simulink model "openloop5012"  (R2022a)
settings: Solver=VariableStepAuto  StartTime=0.0  StopTime=5000  RelTol=1e-3
settings Model: Creator=danie  LastModifiedBy=danie

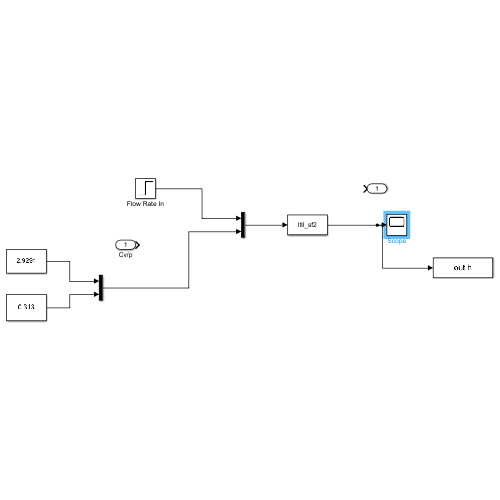
[thumbnail: Simulink's stored preview of the top-level diagram]
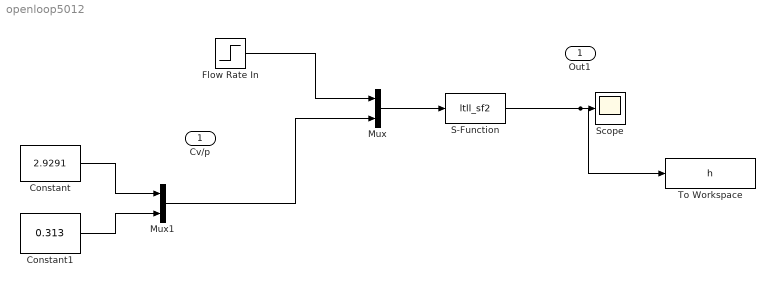
== system openloop5012 ==
  Cv/p : Inport
  Constant : Constant  Value=2.9291
  Constant1 : Constant  Value=0.313
  Flow Rate In : Step  Time=2000  Before=2.5  After=2.7  SampleTime=0
  Mux : Mux  Inputs=2
  Mux1 : Mux  Inputs=2
  S-Function : S-Function  FunctionName=ltll_sf2  SFunctionDeploymentMode=off  EnableBusSupport=off
  Scope : Scope
  To Workspace : ToWorkspace  VariableName=h  SampleTime=-1
  Out1 : Outport
  wires:
  Constant/1 -> Mux1/1
  Flow Rate In/1 -> Mux/1
  Mux/1 -> S-Function/1
  S-Function/1 -> To Workspace/1, Scope/1
  Constant1/1 -> Mux1/2
  Mux1/1 -> Mux/2
